simulink model "Optimization_getVZ"  (R2017b)
settings: Solver=VariableStepAuto  StartTime=0.0  StopTime=Reference_time  RelTol=1e-3
values from neighbouring files (symbols this model uses):
  Ts = plant.Ts    [CoprimeFactorizationSS.m]    (also in ID_Model.m = 0.001; ID_Model_4.m = 0.001; ID_Model_ITRI.m = 0.001; gConstraintFun.m = P.Ts)
undefined symbols (not defined in the file or in its folder): plant
settings Model: Creator=LAB_JHU  LastModifiedBy=LAB_JHU

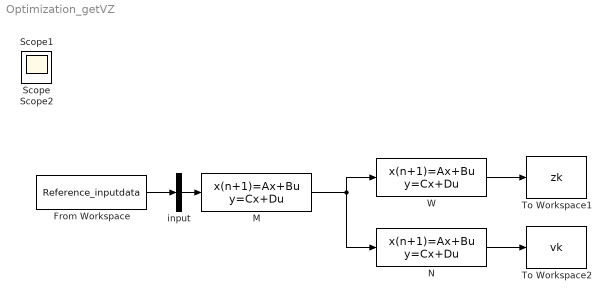
== system Optimization_getVZ ==
  From Workspace : FromWorkspace  VariableName=Reference_inputdata  SampleTime=Ts
  M : DiscreteStateSpace  A=plant.M.A  B=plant.M.B  C=plant.M.C  D=plant.M.D  SampleTime=-1
  N : DiscreteStateSpace  A=plant.N.A  B=plant.N.B  C=plant.N.C  D=plant.N.D  SampleTime=-1
  To Workspace1 : ToWorkspace  VariableName=zk  SampleTime=-1
  To Workspace2 : ToWorkspace  VariableName=vk  SampleTime=-1
  W : DiscreteStateSpace  A=plant.W.A  B=plant.W.B  C=plant.W.C  D=plant.W.D  SampleTime=-1
  input : Demux  Outputs=1
  Scope : Scope
  Scope1 : Scope
  Scope2 : Scope
  wires:
  input/1 -> M/1
  M/1 -> N/1, W/1
  W/1 -> To Workspace1/1
  N/1 -> To Workspace2/1
  From Workspace/1 -> input/1
